simulink model "CAN_TX_RX"  (R2020a)
settings: Solver=FixedStepDiscrete  StartTime=0.0  StopTime=10.0  FixedStep=50e-3  RelTol=1e-3  EnableMultiTasking=on
InitFcn:
  | mbd_s32k_consistency_checks(bdroot(gcs));
undefined symbols (not defined in the file or in its folder): Data, LQFP
libraries: mbd_s32k1xx_ec_toolbox x40, simulink x17, etargetslib x15
(part 1 of 2)
settings Model: Creator=RolandoA  LastModifiedBy=rolan
settings DataIOCC: ExternalInput=off  InitialState=off  SaveOutput=off  SignalLogging=off  SaveTime=off
settings OptimizationCC: DefaultParameterBehavior=Inlined  EnhancedBackFolding=on  PassReuseOutputArgsAs=Individual arguments  ZeroExternalMemoryAtStartup=off  ZeroInternalMemoryAtStartup=off  OptimizeBlockOrder=speed  DifferentSizesBufferReuse=on  OptimizationCustomize=off  EfficientTunableParamExpr=on
settings DebuggingCC: InheritedTsInSrcMsg=none  SingleTaskRateTransMsg=error  ParameterTunabilityLossMsg=error  UnconnectedInputMsg=error  UnconnectedOutputMsg=error  UnconnectedLineMsg=error  UnknownTsInhSupMsg=error
settings HardwareCC: ProdBitPerPointer=32  ProdBitPerSizeT=32  ProdBitPerPtrDiffT=32  ProdLargestAtomicInteger=Long  ProdLargestAtomicFloat=Double  ProdWordSize=32  ProdHWDeviceType=ARM Compatible->ARM Cortex
settings SFSimCC: MATLABDynamicMemAlloc=off
settings RTWCC: Description=Model Based Design Toolbox S32K1xx Code Generation Target  SystemTargetFile=mbd_s32k.tlc  MakeCommand=mbd_s32k_make_rtw COPY_MDLREF_INCLUDES=0  TemplateMakefile=mbd_s32k.tmf  GenerateReport=on  IncludeHyperlinkInReport=on  LaunchReport=on  GenerateTraceInfo=on  GenerateTraceReport=on  GenerateTraceReportSl=on  GenerateTraceReportSf=on  GenerateTraceReportEml=on  GenerateCodeMetricsReport=on  GenerateCodeReplacementReport=on
settings CodeAppCC: ForceParamTrailComments=on  IgnoreCustomStorageClasses=off  OperatorAnnotations=on  SimulinkDataObjDesc=on  SFDataObjDesc=on  InsertBlockDesc=on
settings STFCustomTargetCC: TargetLangStandard=C99 (ISO)  MultiwordLength=256  CombineOutputUpdateFcns=on  ERTCustomFileBanners=on  SupportContinuousTime=off  SupportNonInlinedSFcns=off  RemoveResetFunc=on  MATLABClassNameForMDSCustomization=Simulink.SoftwareTarget.ERTCustomization  SystemTargetFile=mbd_s32k.tlc
settings ERTTargetCC: TargetLangStandard=C99 (ISO)  ParMdlRefBuildCompliant=off  CompOptLevelCompliant=off  ConcurrentExecutionCompliant=off  ModelStepFunctionPrototypeControlCompliant=off  CPPClassGenCompliant=off  UseToolchainInfoCompliant=off  InlinedParameterPlacement=NonHierarchical  ERTSrcFileBannerTemplate=mbd_ert_code_template.cgt  ERTHdrFileBannerTemplate=mbd_ert_code_template.cgt  ERTDataSrcFileTemplate=mbd_ert_code_template.cgt  ERTDataHdrFileTemplate=mbd_ert_code_template.cgt  ERTCustomFileTemplate=example_file_process.tlc

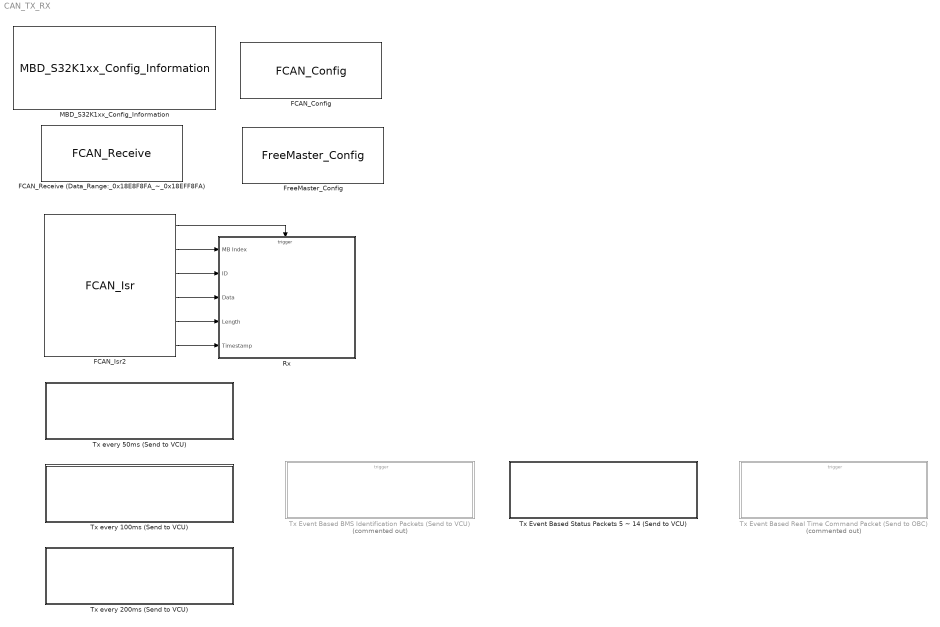
== system CAN_TX_RX ==
  FCAN_Config : mbd_s32k1xx_ec_toolbox/Communication Blocks/CAN Blocks/FCAN_Config  Priority=1  can_instance=0  can_mode=Normal mode  can_max_num_mb=32  can_rx=PTE4: [CAN0_RX | CAN Rx channel]  can_tx=PTE5: [CAN0_TX | CAN Tx Channel]  show_adv_opts=on  can_clk_src=Peripheral clock  bitrate=250  bitrate_adv_opts=off  can_presdiv=15  can_rjw=3  can_pseg1=6  can_pseg2=3  can_propseg=7  can_cbt_presdiv=39  can_cbt_rjw=3  can_cbt_pseg1=5  can_cbt_pseg2=5  can_cbt_propseg=27  can_fd_enable=off  can_payload=8  can_rxfifo_enable=off  can_fifo_id_filter_extended=on  can_fifo_id_filter_remote=off  can_num_id_filters=8  can_fifo_id_format=A  can_fifo_id_filter={'0x0', '0x0', '0x0', '0x0', '0x0', '0x0', '0x0', '0x0'}  can_pn_enable=off  can_wakeup_match=off  can_wakeup_timeout=off  can_timeout_en=off  can_match_timeout=1  can_multiple_matches_en=off  can_num_matches=1  can_idfilter_extendedid=off  can_idfilter_remoteframe=off  can_idfilter_type=Match exact  can_idfilter_id1=0  can_idfilter_id2=0  can_payloadfilter_enable=off  can_payloadfilter_dlclow=0  can_payloadfilter_dlchigh=0  can_payloadfilter_type=Match exact  can_payloadfilter_payload1_b0=0  can_payloadfilter_payload1_b1=0  can_payloadfilter_payload1_b2=0  can_payloadfilter_payload1_b3=0  can_payloadfilter_payload1_b4=0  can_payloadfilter_payload1_b5=0  can_payloadfilter_payload1_b6=0  can_payloadfilter_payload1_b7=0  can_payloadfilter_payload2_b0=0  can_payloadfilter_payload2_b1=0  can_payloadfilter_payload2_b2=0  can_payloadfilter_payload2_b3=0  can_payloadfilter_payload2_b4=0  can_payloadfilter_payload2_b5=0  can_payloadfilter_payload2_b6=0  can_payloadfilter_payload2_b7=0
  FCAN_Isr2 : mbd_s32k1xx_ec_toolbox/Communication Blocks/CAN Blocks/FCAN_Isr  can_instance=0  can_event=Rx Complete
  FCAN_Receive (Data_Range:_0x18E8F8FA_~_0x18EFF8FA) : mbd_s32k1xx_ec_toolbox/Communication Blocks/CAN Blocks/FCAN_Receive  can_instance=0  can_mode=Non-blocking  can_timeout_ms=0  can_mb_idx=0  can_extended_id=on  can_is_remote=off  can_id=18E8F8FA  can_msg_mask=FFF8FFFF  show_adv_opts=on  can_use_rxfifo=off  can_fd_enable=off
  FreeMaster_Config : mbd_s32k1xx_ec_toolbox/Utility Blocks/FreeMaster_Config  interface=LPUART1  baudrate=115200  rxd=PTC6: [LPUART1_RX | Receive]  txd=PTC7: [LPUART1_TX | Transmit]  mode=Poll-driven  isr_prio=15  show_adv_opts=on  use_scope=on  max_scope_vars=8  use_recorder=on  max_rec_vars=8  rec_buff_size=1024  rec_timebase=0 seconds  comm_buffer_size_auto=on  comm_buffer_size=255  comm_rqueue_size_default=on  comm_rqueue_size=32
  MBD_S32K1xx_Config_Information : mbd_s32k1xx_ec_toolbox/MBD_S32K1xx_Config_Information  mbdt_ver=0  disp_str=|  config_params=[]  mcu_target_name=S32K144  mcu_target_package=100-LQFP  mcu_target_sram_size=64KB  mcu_system_clock_freq=80  mcu_xtal_freq=External 8  mcu_steptick_timer=LPIT Channel 0  mcu_steptick_prio=15  ds_import_enable=on  target_compiler=GCC  target_memory=FLASH  gcc_target_compile_opts=-mthumb -mfloat-abi=hard -mfpu=fpv4-sp-d16 -O1 -g -gstrict-dwarf  gcc_target_assemble_opts=-mthumb -mfloat-abi=hard -mfpu=fpv4-sp-d16 -g  gcc_target_link_opts=-mthumb -mfloat-abi=hard -mfpu=fpv4-sp-d16  gcc_target_default_lcf=on  gcc_target_user_lcf=S32K148_192_flash.ld  ghs_target_compile_opts=-cpu=cortexm4f -thumb -fpu=vfpv4_d16 -fsingle -Ogeneral -Wundef -Wimplicit-int -Wshadow -Wtrigraphs --no_commons --gnu_asm -gnu99 -gdwarf-2 -G  ghs_target_assemble_opts=-cpu=cortexm4f -fpu=vfpv4_d16  ghs_target_link_opts=-cpu=cortexm4f -thumb -fpu=vfpv4_d16  ghs_target_default_lcf=on  ghs_target_user_lcf=S32K148_192_flash.ld  iar_target_compile_opts=--cpu=Cortex-M4F --thumb --fpu=VFPv4_sp -Ol -e --debug --dlib_config normal  iar_target_assemble_opts=--cpu Cortex-M4F --thumb --fpu VFPv4_sp  iar_target_link_opts=--no_exceptions --vfe --inline  iar_target_default_lcf=on  iar_target_user_lcf=S32K148_192_flash.icf  pil_download_enable=off  rbl_download_enable=on  rbl_start_delay=5000  rbl_download_interface=OpenSDA  rbl_restart_request=off  rbl_com_port=Custom  rbl_com_port_custom=COM1  pil_download_rate=57600  pil_opensda_drive=Custom  pil_opensda_drive_custom=D  pil_uart_instance=1  pil_uart_rx=PTC6: [LPUART1_RX | Receive]  pil_uart_tx=PTC7: [LPUART1_TX | Transmit]  FTM_PWM_PcrCheckEnDis=on  FTM_Input_Edge_Inputs_PcrCheckEnDis=on  FTM_Dual_Edge_Inputs_PcrCheckEnDis=on  FTM_Quadrature_Inputs_PcrCheckEnDis=on  FTM_Hall_Sensor_Inputs_PcrCheckEnDis=on  LPTMR_PcrCheckEnDis=on  PIT_PcrCheckEnDis=on  RTC_PcrCheckEnDis=on  FlexCAN_PcrCheckEnDis=on  LIN_PcrCheckEnDis=on  FlexIO_PcrCheckEnDis=on  LPI2C_PcrCheckEnDis=on  LPSPI_PcrCheckEnDis=on  LPUART_PcrCheckEnDis=on  CMP_PcrCheckEnDis=on  GPIO_OutputPcrCheckEnDis=on  GPIO_InputPcrCheckEnDis=on  SBC_PcrCheckEnDis=on  BMS_PcrCheckEnDis=on  AMMCLIB_PcrCheckEnDis=on  FM_PcrCheckEnDis=on  Profile_PcrCheckEnDis=on  ConfigParams_PcrCheckEnDis=on  ModelRef_PcrCheckEnDis=on  PDB0_PcrCheckEnDis=on  CSEc_PcrCheckEnDis=on  eDMA_PcrCheckEnDis=on  FLASH_PcrCheckEnDis=on  ADC_PcrCheckEnDis=on  WDOG_PcrCheckEnDis=on
      | Target : S32K144-64KB_SRAM
      | Package : 100-pin
      | System clock : 80 MHz
      | XTAL clock : External 8 MHz
      | Compiler : IAR
      | Target Type : FLASH
      | Download Code after build : off
      | Step Tick Interrupt Priority : 15
  Rx : Subsystem  TreatAsAtomicUnit=on
  "Tx Event Based BMS Identification Packets (Send to VCU)   " : Subsystem  Commented=on  TreatAsAtomicUnit=on
  Tx Event Based Real Time Command Packet (Send to OBC) : Subsystem  Commented=on  TreatAsAtomicUnit=on
  Tx Event Based Status Packets 5 ~ 14 (Send to VCU) : Subsystem  TreatAsAtomicUnit=on
  Tx every 100ms (Send to VCU) : Subsystem  TreatAsAtomicUnit=on  SystemSampleTime=100e-3
  Tx every 200ms (Send to VCU) : Subsystem  TreatAsAtomicUnit=on  SystemSampleTime=200e-3
  Tx every 50ms (Send to VCU) : Subsystem  TreatAsAtomicUnit=on  SystemSampleTime=50e-3
  wires:
  FCAN_Isr2/1 -> Rx/Trigger
  FCAN_Isr2/2 -> Rx/1(MB Index)
  FCAN_Isr2/3 -> Rx/2(ID)
  FCAN_Isr2/4 -> Rx/3(Data)
  FCAN_Isr2/5 -> Rx/4(Length)
  FCAN_Isr2/6 -> Rx/5(Timestamp)

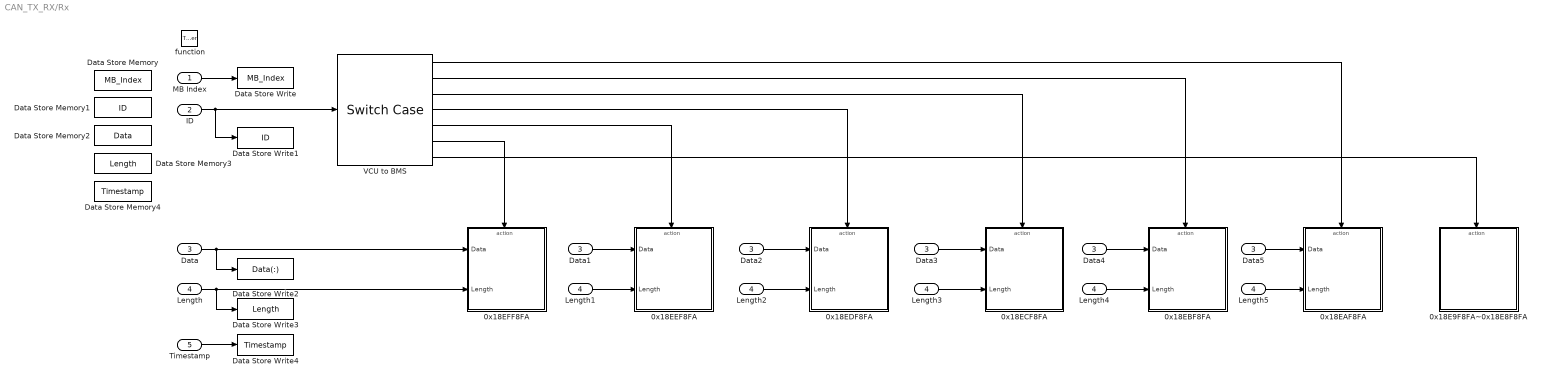
== system CAN_TX_RX/Rx ==
  MB Index : Inport
  ID : Inport  Port=2
  Data : Inport  Port=3
  Length : Inport  Port=4
  Timestamp : Inport  Port=5
  function : TriggerPort  TriggerType=function-call  VariantControl=Variant
  0x18E9F8FA~0x18E8F8FA : Subsystem  TreatAsAtomicUnit=on
  0x18EAF8FA : Subsystem  TreatAsAtomicUnit=on
  0x18EBF8FA : Subsystem  TreatAsAtomicUnit=on
  0x18ECF8FA : Subsystem  TreatAsAtomicUnit=on
  0x18EDF8FA : Subsystem  TreatAsAtomicUnit=on
  0x18EEF8FA : Subsystem  TreatAsAtomicUnit=on
  0x18EFF8FA : Subsystem  TreatAsAtomicUnit=on
  Data Store Memory : DataStoreMemory  DataStoreName=MB_Index  ReadBeforeWriteMsg=warning  WriteAfterWriteMsg=warning  WriteAfterReadMsg=warning  ShowAdditionalParam=off  OutDataTypeStr=uint8
  Data Store Memory1 : DataStoreMemory  DataStoreName=ID  ReadBeforeWriteMsg=warning  WriteAfterWriteMsg=warning  WriteAfterReadMsg=warning  ShowAdditionalParam=off  OutDataTypeStr=uint32
  Data Store Memory2 : DataStoreMemory  DataStoreName=Data  ReadBeforeWriteMsg=warning  WriteAfterWriteMsg=warning  WriteAfterReadMsg=warning  InitialValue=[0 0 0 0 0 0 0 0]  ShowAdditionalParam=off  OutDataTypeStr=uint8
  Data Store Memory3 : DataStoreMemory  DataStoreName=Length  ReadBeforeWriteMsg=warning  WriteAfterWriteMsg=warning  WriteAfterReadMsg=warning  ShowAdditionalParam=off  OutDataTypeStr=uint8
  Data Store Memory4 : DataStoreMemory  DataStoreName=Timestamp  ReadBeforeWriteMsg=warning  WriteAfterWriteMsg=warning  WriteAfterReadMsg=warning  ShowAdditionalParam=off  OutDataTypeStr=uint16
  Data Store Write : DataStoreWrite  DataStoreName=MB_Index
  Data Store Write1 : DataStoreWrite  DataStoreName=ID
  Data Store Write2 : DataStoreWrite  DataStoreName=Data  DataStoreElements=Data(:)
  Data Store Write3 : DataStoreWrite  DataStoreName=Length
  Data Store Write4 : DataStoreWrite  DataStoreName=Timestamp
  Data{1..5} (5 alike) : InportShadow  Port=3
  Length{1..5} (5 alike) : InportShadow  Port=4
  VCU to BMS : SwitchCase  CaseConditions={418052346, 418117882, 418183418, 418248954, 418314490, 418380026}
  wires:
  MB Index/1 -> Data Store Write/1
  ID/1 -> VCU to BMS/1, Data Store Write1/1
  Data/1 -> Data Store Write2/1, 0x18EFF8FA/1(Data)
  Length/1 -> Data Store Write3/1, 0x18EFF8FA/2(Length)
  Timestamp/1 -> Data Store Write4/1
  VCU to BMS/7 -> 0x18E9F8FA~0x18E8F8FA/Action
  VCU to BMS/6 -> 0x18EFF8FA/Action
  VCU to BMS/2 -> 0x18EBF8FA/Action
  VCU to BMS/3 -> 0x18ECF8FA/Action
  VCU to BMS/4 -> 0x18EDF8FA/Action
  VCU to BMS/5 -> 0x18EEF8FA/Action
  Data1/1 -> 0x18EEF8FA/1(Data)
  Length1/1 -> 0x18EEF8FA/2(Length)
  Data2/1 -> 0x18EDF8FA/1(Data)
  Length2/1 -> 0x18EDF8FA/2(Length)
  Length3/1 -> 0x18ECF8FA/2(Length)
  Data3/1 -> 0x18ECF8FA/1(Data)
  Data4/1 -> 0x18EBF8FA/1(Data)
  Length4/1 -> 0x18EBF8FA/2(Length)
  VCU to BMS/1 -> 0x18EAF8FA/Action
  Data5/1 -> 0x18EAF8FA/1(Data)
  Length5/1 -> 0x18EAF8FA/2(Length)

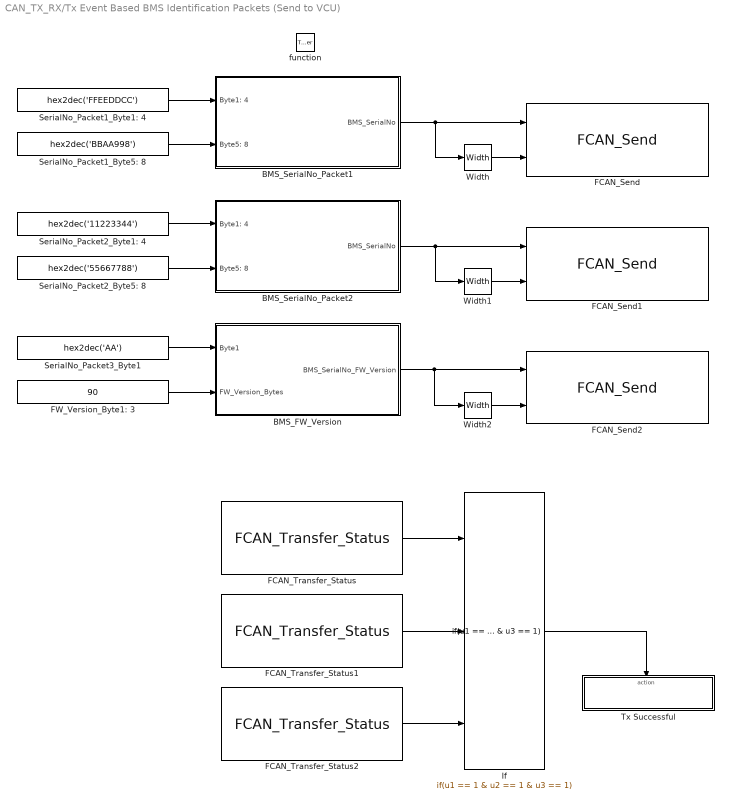
== system CAN_TX_RX/Tx Event Based BMS Identification Packets (Send to VCU)    ==
  function : TriggerPort  TriggerType=function-call  VariantControl=Variant
  BMS_FW_Version : Subsystem
  BMS_SerialNo_Packet1 : Subsystem
  BMS_SerialNo_Packet2 : Subsystem
  FCAN_Send : mbd_s32k1xx_ec_toolbox/Communication Blocks/CAN Blocks/FCAN_Send  can_instance=0  can_mode=Non-blocking  can_timeout_ms=0  can_mb_idx=5  can_extended_id=on  can_is_remote=off  can_id=18EBFAF8  show_adv_opts=on  can_fd_enable=off  can_enable_brs=off  can_fd_padding=0
  FCAN_Send1 : mbd_s32k1xx_ec_toolbox/Communication Blocks/CAN Blocks/FCAN_Send  can_instance=0  can_mode=Non-blocking  can_timeout_ms=0  can_mb_idx=6  can_extended_id=on  can_is_remote=off  can_id=18EAFAF8  show_adv_opts=on  can_fd_enable=off  can_enable_brs=off  can_fd_padding=0
  FCAN_Send2 : mbd_s32k1xx_ec_toolbox/Communication Blocks/CAN Blocks/FCAN_Send  can_instance=0  can_mode=Non-blocking  can_timeout_ms=0  can_mb_idx=7  can_extended_id=on  can_is_remote=off  can_id=18E9FAF8  show_adv_opts=on  can_fd_enable=off  can_enable_brs=off  can_fd_padding=0
  FCAN_Transfer_Status : mbd_s32k1xx_ec_toolbox/Communication Blocks/CAN Blocks/FCAN_Transfer_Status  can_instance=0  can_mb_idx=5
  FCAN_Transfer_Status1 : mbd_s32k1xx_ec_toolbox/Communication Blocks/CAN Blocks/FCAN_Transfer_Status  can_instance=0  can_mb_idx=6
  FCAN_Transfer_Status2 : mbd_s32k1xx_ec_toolbox/Communication Blocks/CAN Blocks/FCAN_Transfer_Status  can_instance=0  can_mb_idx=7
  FW_Version_Byte1: 3 : Constant  Value=90  OutDataTypeStr=uint32
  If : If  NumInputs=3  IfExpression=u1 == 1 & u2 == 1 & u3 == 1  ShowElse=off
  SerialNo_Packet1_Byte1: 4 : Constant  Value=hex2dec('FFEEDDCC')  OutDataTypeStr=uint32
  SerialNo_Packet1_Byte5: 8 : Constant  Value=hex2dec('BBAA998')  OutDataTypeStr=uint32
  SerialNo_Packet2_Byte1: 4 : Constant  Value=hex2dec('11223344')  OutDataTypeStr=uint32
  SerialNo_Packet2_Byte5: 8 : Constant  Value=hex2dec('55667788')  OutDataTypeStr=uint32
  SerialNo_Packet3_Byte1 : Constant  Value=hex2dec('AA')  OutDataTypeStr=uint8
  Tx Successful : Subsystem  TreatAsAtomicUnit=on
  Width : Width  DataType=uint8
  Width1 : Width  DataType=uint8
  Width2 : Width  DataType=uint8
  wires:
  BMS_SerialNo_Packet1/1(BMS_SerialNo) -> Width/1, FCAN_Send/1
  Width/1 -> FCAN_Send/2
  FCAN_Transfer_Status/1 -> If/1
  FCAN_Transfer_Status1/1 -> If/2
  FCAN_Transfer_Status2/1 -> If/3
  If/1 -> Tx Successful/Action
  Width1/1 -> FCAN_Send1/2
  Width2/1 -> FCAN_Send2/2
  SerialNo_Packet1_Byte1: 4/1 -> BMS_SerialNo_Packet1/1(Byte1: 4)
  SerialNo_Packet1_Byte5: 8/1 -> BMS_SerialNo_Packet1/2(Byte5: 8)
  SerialNo_Packet2_Byte1: 4/1 -> BMS_SerialNo_Packet2/1(Byte1: 4)
  SerialNo_Packet2_Byte5: 8/1 -> BMS_SerialNo_Packet2/2(Byte5: 8)
  BMS_SerialNo_Packet2/1(BMS_SerialNo) -> Width1/1, FCAN_Send1/1
  SerialNo_Packet3_Byte1/1 -> BMS_FW_Version/1(Byte1)
  FW_Version_Byte1: 3/1 -> BMS_FW_Version/2(FW_Version_Bytes)
  BMS_FW_Version/1(BMS_SerialNo_FW_Version) -> Width2/1, FCAN_Send2/1

== system CAN_TX_RX/Tx Event Based Real Time Command Packet (Send to OBC) ==
  function : TriggerPort  TriggerType=function-call  VariantControl=Variant
  FCAN_Send : mbd_s32k1xx_ec_toolbox/Communication Blocks/CAN Blocks/FCAN_Send  Commented=on  can_instance=0  can_mode=Non-blocking  can_timeout_ms=0  can_mb_idx=18  can_extended_id=on  can_is_remote=off  can_id=18EFF2F8  show_adv_opts=on  can_fd_enable=off  can_enable_brs=off  can_fd_padding=0
  FCAN_Transfer_Status : mbd_s32k1xx_ec_toolbox/Communication Blocks/CAN Blocks/FCAN_Transfer_Status  Commented=on  can_instance=0  can_mb_idx=18
  If : If  Commented=on  IfExpression=u1 == 1  ShowElse=off
  Tx Successful : Subsystem  Commented=on  TreatAsAtomicUnit=on
  wires:
  FCAN_Transfer_Status/1 -> If/1
  If/1 -> Tx Successful/Action

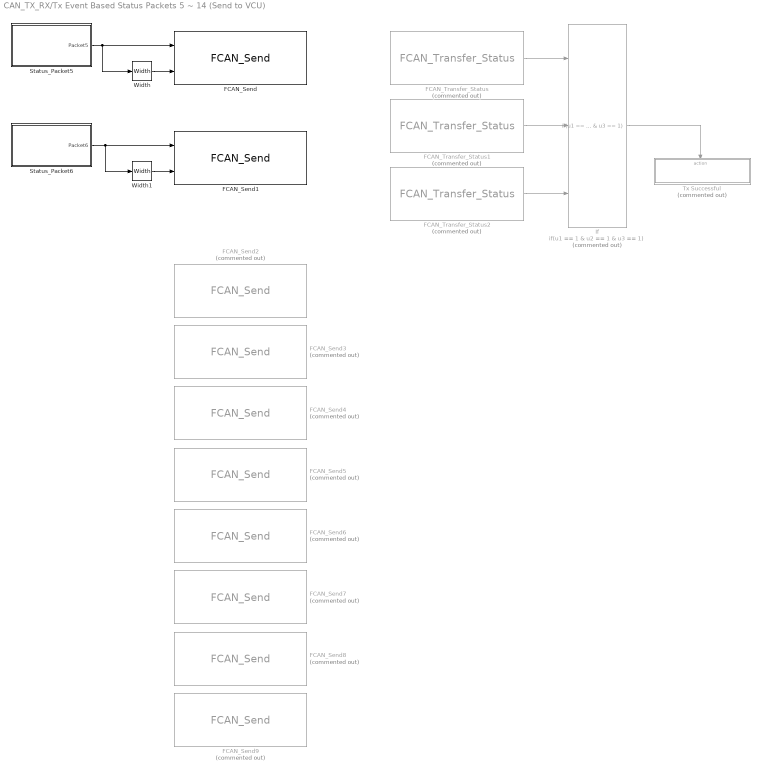
== system CAN_TX_RX/Tx Event Based Status Packets 5 ~ 14 (Send to VCU) ==
  FCAN_Send : mbd_s32k1xx_ec_toolbox/Communication Blocks/CAN Blocks/FCAN_Send  can_instance=0  can_mode=Non-blocking  can_timeout_ms=0  can_mb_idx=8  can_extended_id=on  can_is_remote=off  can_id=18E8FAF8  show_adv_opts=on  can_fd_enable=off  can_enable_brs=off  can_fd_padding=0
  FCAN_Send1 : mbd_s32k1xx_ec_toolbox/Communication Blocks/CAN Blocks/FCAN_Send  can_instance=0  can_mode=Non-blocking  can_timeout_ms=0  can_mb_idx=9  can_extended_id=on  can_is_remote=off  can_id=18E7FAF8  show_adv_opts=on  can_fd_enable=off  can_enable_brs=off  can_fd_padding=0
  FCAN_Send2 : mbd_s32k1xx_ec_toolbox/Communication Blocks/CAN Blocks/FCAN_Send  Commented=on  can_instance=0  can_mode=Non-blocking  can_timeout_ms=0  can_mb_idx=10  can_extended_id=on  can_is_remote=off  can_id=18E6FAF8  show_adv_opts=on  can_fd_enable=off  can_enable_brs=off  can_fd_padding=0
  FCAN_Send3 : mbd_s32k1xx_ec_toolbox/Communication Blocks/CAN Blocks/FCAN_Send  Commented=on  can_instance=0  can_mode=Non-blocking  can_timeout_ms=0  can_mb_idx=11  can_extended_id=on  can_is_remote=off  can_id=18E5FAF8  show_adv_opts=on  can_fd_enable=off  can_enable_brs=off  can_fd_padding=0
  FCAN_Send4 : mbd_s32k1xx_ec_toolbox/Communication Blocks/CAN Blocks/FCAN_Send  Commented=on  can_instance=0  can_mode=Non-blocking  can_timeout_ms=0  can_mb_idx=12  can_extended_id=on  can_is_remote=off  can_id=18E4FAF8  show_adv_opts=on  can_fd_enable=off  can_enable_brs=off  can_fd_padding=0
  FCAN_Send5 : mbd_s32k1xx_ec_toolbox/Communication Blocks/CAN Blocks/FCAN_Send  Commented=on  can_instance=0  can_mode=Non-blocking  can_timeout_ms=0  can_mb_idx=13  can_extended_id=on  can_is_remote=off  can_id=18E3FAF8  show_adv_opts=on  can_fd_enable=off  can_enable_brs=off  can_fd_padding=0
  FCAN_Send6 : mbd_s32k1xx_ec_toolbox/Communication Blocks/CAN Blocks/FCAN_Send  Commented=on  can_instance=0  can_mode=Non-blocking  can_timeout_ms=0  can_mb_idx=14  can_extended_id=on  can_is_remote=off  can_id=18E2FAF8  show_adv_opts=on  can_fd_enable=off  can_enable_brs=off  can_fd_padding=0
  FCAN_Send7 : mbd_s32k1xx_ec_toolbox/Communication Blocks/CAN Blocks/FCAN_Send  Commented=on  can_instance=0  can_mode=Non-blocking  can_timeout_ms=0  can_mb_idx=15  can_extended_id=on  can_is_remote=off  can_id=18E1FAF8  show_adv_opts=on  can_fd_enable=off  can_enable_brs=off  can_fd_padding=0
  FCAN_Send8 : mbd_s32k1xx_ec_toolbox/Communication Blocks/CAN Blocks/FCAN_Send  Commented=on  can_instance=0  can_mode=Non-blocking  can_timeout_ms=0  can_mb_idx=16  can_extended_id=on  can_is_remote=off  can_id=18E0FAF8  show_adv_opts=on  can_fd_enable=off  can_enable_brs=off  can_fd_padding=0
  FCAN_Send9 : mbd_s32k1xx_ec_toolbox/Communication Blocks/CAN Blocks/FCAN_Send  Commented=on  can_instance=0  can_mode=Non-blocking  can_timeout_ms=0  can_mb_idx=17  can_extended_id=on  can_is_remote=off  can_id=18DFFAF8  show_adv_opts=on  can_fd_enable=off  can_enable_brs=off  can_fd_padding=0
  FCAN_Transfer_Status : mbd_s32k1xx_ec_toolbox/Communication Blocks/CAN Blocks/FCAN_Transfer_Status  Commented=on  can_instance=0  can_mb_idx=5
  FCAN_Transfer_Status1 : mbd_s32k1xx_ec_toolbox/Communication Blocks/CAN Blocks/FCAN_Transfer_Status  Commented=on  can_instance=0  can_mb_idx=6
  FCAN_Transfer_Status2 : mbd_s32k1xx_ec_toolbox/Communication Blocks/CAN Blocks/FCAN_Transfer_Status  Commented=on  can_instance=0  can_mb_idx=7
  If : If  Commented=on  NumInputs=3  IfExpression=u1 == 1 & u2 == 1 & u3 == 1  ShowElse=off
  Status_Packet5 : Subsystem
  Status_Packet6 : Subsystem
  Tx Successful : Subsystem  Commented=on  TreatAsAtomicUnit=on
  Width : Width  DataType=uint8
  Width1 : Width  DataType=uint8
  wires:
  If/1 -> Tx Successful/Action
  FCAN_Transfer_Status2/1 -> If/3
  FCAN_Transfer_Status1/1 -> If/2
  FCAN_Transfer_Status/1 -> If/1
  Status_Packet5/1(Packet5) -> FCAN_Send/1, Width/1
  Width/1 -> FCAN_Send/2
  Width1/1 -> FCAN_Send1/2
  Status_Packet6/1(Packet6) -> Width1/1, FCAN_Send1/1

== system CAN_TX_RX/Tx every 100ms (Send to VCU) ==
  FCAN_Send : mbd_s32k1xx_ec_toolbox/Communication Blocks/CAN Blocks/FCAN_Send  can_instance=0  can_mode=Non-blocking  can_timeout_ms=0  can_mb_idx=4  can_extended_id=on  can_is_remote=off  can_id=18ECFAF8  show_adv_opts=on  can_fd_enable=off  can_enable_brs=off  can_fd_padding=0
  FCAN_Transfer_Status : mbd_s32k1xx_ec_toolbox/Communication Blocks/CAN Blocks/FCAN_Transfer_Status  can_instance=0  can_mb_idx=4
  If : If  IfExpression=u1 == 1  ShowElse=off
  Status_Packet4 : Subsystem
  Tx Succesful : Subsystem  TreatAsAtomicUnit=on
  Width : Width  DataType=uint8
  wires:
  Width/1 -> FCAN_Send/2
  Status_Packet4/1(Packet4) -> FCAN_Send/1, Width/1
  If/1 -> Tx Succesful/Action
  FCAN_Transfer_Status/1 -> If/1

== system CAN_TX_RX/Tx every 200ms (Send to VCU) ==
  FCAN_Send : mbd_s32k1xx_ec_toolbox/Communication Blocks/CAN Blocks/FCAN_Send  can_instance=0  can_mode=Non-blocking  can_timeout_ms=0  can_mb_idx=2  can_extended_id=on  can_is_remote=off  can_id=18EEFAF8  show_adv_opts=on  can_fd_enable=off  can_enable_brs=off  can_fd_padding=0
  FCAN_Send1 : mbd_s32k1xx_ec_toolbox/Communication Blocks/CAN Blocks/FCAN_Send  can_instance=0  can_mode=Non-blocking  can_timeout_ms=0  can_mb_idx=3  can_extended_id=on  can_is_remote=off  can_id=18EDFAF8  show_adv_opts=on  can_fd_enable=off  can_enable_brs=off  can_fd_padding=0
  FCAN_Transfer_Status : mbd_s32k1xx_ec_toolbox/Communication Blocks/CAN Blocks/FCAN_Transfer_Status  can_instance=0  can_mb_idx=2
  FCAN_Transfer_Status1 : mbd_s32k1xx_ec_toolbox/Communication Blocks/CAN Blocks/FCAN_Transfer_Status  can_instance=0  can_mb_idx=3
  If : If  NumInputs=2  IfExpression=u1 == 1 & u2 == 1  ShowElse=off
  Status_Packet2 : Subsystem
  Status_Packet3 : Subsystem
  Tx Successful : Subsystem  TreatAsAtomicUnit=on
  Width : Width  DataType=uint8
  Width1 : Width  DataType=uint8
  wires:
  Width/1 -> FCAN_Send/2
  Status_Packet2/1(Packet2) -> FCAN_Send/1, Width/1
  If/1 -> Tx Successful/Action
  FCAN_Transfer_Status/1 -> If/1
  Width1/1 -> FCAN_Send1/2
  Status_Packet3/1(Packet3) -> Width1/1, FCAN_Send1/1
  FCAN_Transfer_Status1/1 -> If/2

== system CAN_TX_RX/Tx every 50ms (Send to VCU) ==
  FCAN_Send : mbd_s32k1xx_ec_toolbox/Communication Blocks/CAN Blocks/FCAN_Send  can_instance=0  can_mode=Non-blocking  can_timeout_ms=0  can_mb_idx=1  can_extended_id=on  can_is_remote=off  can_id=18EFFAF8  show_adv_opts=on  can_fd_enable=off  can_enable_brs=off  can_fd_padding=0
  FCAN_Transfer_Status : mbd_s32k1xx_ec_toolbox/Communication Blocks/CAN Blocks/FCAN_Transfer_Status  can_instance=0  can_mb_idx=1
  If : If  IfExpression=u1 == 1  ShowElse=off
  Status_Packet1 : Subsystem
  Tx Succesful : Subsystem  TreatAsAtomicUnit=on
  Width : Width  DataType=uint8
  wires:
  FCAN_Transfer_Status/1 -> If/1
  If/1 -> Tx Succesful/Action
  Status_Packet1/1(Packet1) -> Width/1, FCAN_Send/1
  Width/1 -> FCAN_Send/2

== system CAN_TX_RX/Rx/0x18E9F8FA~0x18E8F8FA ==
  Action Port : ActionPort  ActionPortLabel=default:

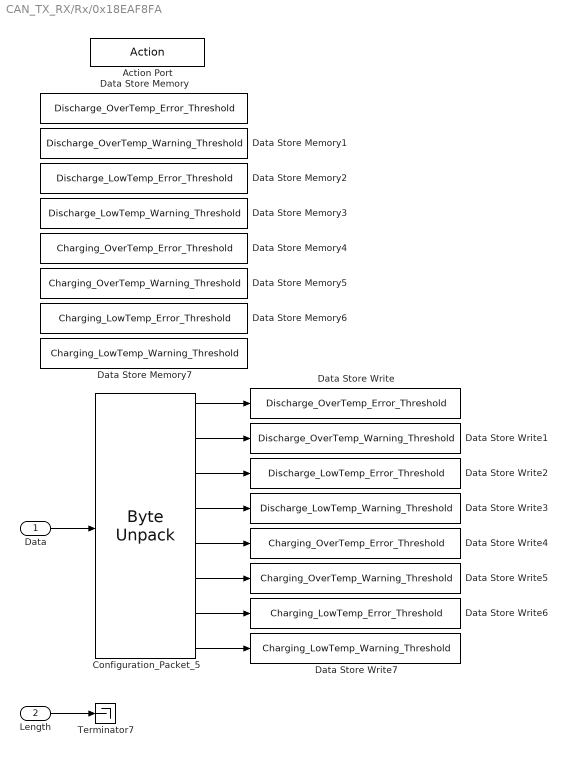
== system CAN_TX_RX/Rx/0x18EAF8FA ==
  Data : Inport
  Length : Inport  Port=2
  Action Port : ActionPort  ActionPortLabel=case [ 418052346 ]:
  Configuration_Packet_5 : etargetslib/Byte Unpack  dimensions={1, 1, 1, 1, 1, 1, 1, 1}  datatypes={'uint8', 'uint8', 'uint8', 'uint8', 'uint8', 'uint8', 'uint8', 'uint8'}  byteAlign=1
  Data Store Memory : DataStoreMemory  DataStoreName=Discharge_OverTemp_Error_Threshold  ReadBeforeWriteMsg=warning  WriteAfterWriteMsg=warning  WriteAfterReadMsg=warning  ShowAdditionalParam=off
  Data Store Memory1 : DataStoreMemory  DataStoreName=Discharge_OverTemp_Warning_Threshold  ReadBeforeWriteMsg=warning  WriteAfterWriteMsg=warning  WriteAfterReadMsg=warning  ShowAdditionalParam=off
  Data Store Memory2 : DataStoreMemory  DataStoreName=Discharge_LowTemp_Error_Threshold  ReadBeforeWriteMsg=warning  WriteAfterWriteMsg=warning  WriteAfterReadMsg=warning  ShowAdditionalParam=off
  Data Store Memory3 : DataStoreMemory  DataStoreName=Discharge_LowTemp_Warning_Threshold  ReadBeforeWriteMsg=warning  WriteAfterWriteMsg=warning  WriteAfterReadMsg=warning  ShowAdditionalParam=off
  Data Store Memory4 : DataStoreMemory  DataStoreName=Charging_OverTemp_Error_Threshold  ReadBeforeWriteMsg=warning  WriteAfterWriteMsg=warning  WriteAfterReadMsg=warning  ShowAdditionalParam=off
  Data Store Memory5 : DataStoreMemory  DataStoreName=Charging_OverTemp_Warning_Threshold  ReadBeforeWriteMsg=warning  WriteAfterWriteMsg=warning  WriteAfterReadMsg=warning  ShowAdditionalParam=off
  Data Store Memory6 : DataStoreMemory  DataStoreName=Charging_LowTemp_Error_Threshold  ReadBeforeWriteMsg=warning  WriteAfterWriteMsg=warning  WriteAfterReadMsg=warning  ShowAdditionalParam=off
  Data Store Memory7 : DataStoreMemory  DataStoreName=Charging_LowTemp_Warning_Threshold  ReadBeforeWriteMsg=warning  WriteAfterWriteMsg=warning  WriteAfterReadMsg=warning  ShowAdditionalParam=off
  Data Store Write : DataStoreWrite  DataStoreName=Discharge_OverTemp_Error_Threshold
  Data Store Write1 : DataStoreWrite  DataStoreName=Discharge_OverTemp_Warning_Threshold
  Data Store Write2 : DataStoreWrite  DataStoreName=Discharge_LowTemp_Error_Threshold
  Data Store Write3 : DataStoreWrite  DataStoreName=Discharge_LowTemp_Warning_Threshold
  Data Store Write4 : DataStoreWrite  DataStoreName=Charging_OverTemp_Error_Threshold
  Data Store Write5 : DataStoreWrite  DataStoreName=Charging_OverTemp_Warning_Threshold
  Data Store Write6 : DataStoreWrite  DataStoreName=Charging_LowTemp_Error_Threshold
  Data Store Write7 : DataStoreWrite  DataStoreName=Charging_LowTemp_Warning_Threshold
  Terminator7 : Terminator
  wires:
  Data/1 -> Configuration_Packet_5/1
  Length/1 -> Terminator7/1
  Configuration_Packet_5/1 -> Data Store Write/1
  Configuration_Packet_5/2 -> Data Store Write1/1
  Configuration_Packet_5/3 -> Data Store Write2/1
  Configuration_Packet_5/4 -> Data Store Write3/1
  Configuration_Packet_5/5 -> Data Store Write4/1
  Configuration_Packet_5/6 -> Data Store Write5/1
  Configuration_Packet_5/7 -> Data Store Write6/1
  Configuration_Packet_5/8 -> Data Store Write7/1

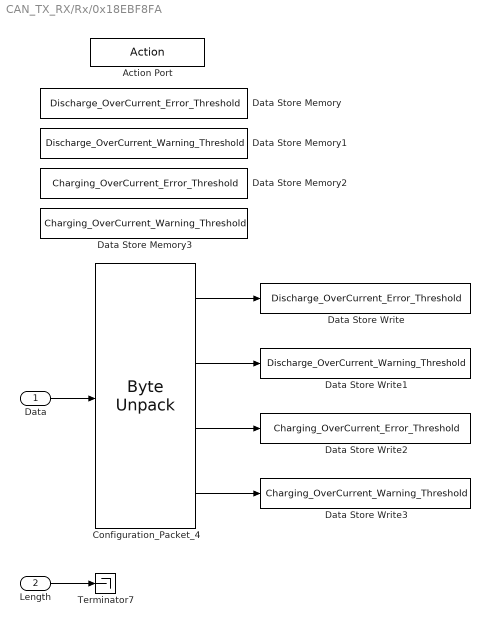
== system CAN_TX_RX/Rx/0x18EBF8FA ==
  Data : Inport
  Length : Inport  Port=2
  Action Port : ActionPort  ActionPortLabel=case [ 418117882 ]:
  Configuration_Packet_4 : etargetslib/Byte Unpack  dimensions={1, 1, 1, 1}  datatypes={'uint16', 'uint16', 'uint16', 'uint16'}  byteAlign=1
  Data Store Memory : DataStoreMemory  DataStoreName=Discharge_OverCurrent_Error_Threshold  ReadBeforeWriteMsg=warning  WriteAfterWriteMsg=warning  WriteAfterReadMsg=warning  ShowAdditionalParam=off
  Data Store Memory1 : DataStoreMemory  DataStoreName=Discharge_OverCurrent_Warning_Threshold  ReadBeforeWriteMsg=warning  WriteAfterWriteMsg=warning  WriteAfterReadMsg=warning  ShowAdditionalParam=off
  Data Store Memory2 : DataStoreMemory  DataStoreName=Charging_OverCurrent_Error_Threshold  ReadBeforeWriteMsg=warning  WriteAfterWriteMsg=warning  WriteAfterReadMsg=warning  ShowAdditionalParam=off
  Data Store Memory3 : DataStoreMemory  DataStoreName=Charging_OverCurrent_Warning_Threshold  ReadBeforeWriteMsg=warning  WriteAfterWriteMsg=warning  WriteAfterReadMsg=warning  ShowAdditionalParam=off
  Data Store Write : DataStoreWrite  DataStoreName=Discharge_OverCurrent_Error_Threshold
  Data Store Write1 : DataStoreWrite  DataStoreName=Discharge_OverCurrent_Warning_Threshold
  Data Store Write2 : DataStoreWrite  DataStoreName=Charging_OverCurrent_Error_Threshold
  Data Store Write3 : DataStoreWrite  DataStoreName=Charging_OverCurrent_Warning_Threshold
  Terminator7 : Terminator
  wires:
  Length/1 -> Terminator7/1
  Data/1 -> Configuration_Packet_4/1
  Configuration_Packet_4/1 -> Data Store Write/1
  Configuration_Packet_4/2 -> Data Store Write1/1
  Configuration_Packet_4/3 -> Data Store Write2/1
  Configuration_Packet_4/4 -> Data Store Write3/1

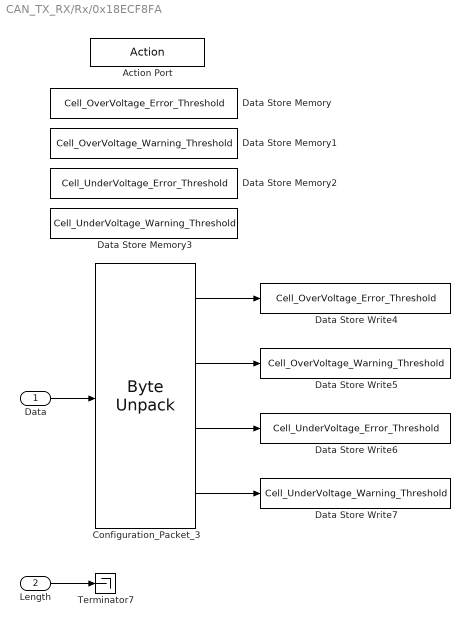
== system CAN_TX_RX/Rx/0x18ECF8FA ==
  Data : Inport
  Length : Inport  Port=2
  Action Port : ActionPort  ActionPortLabel=case [ 418183418 ]:
  Configuration_Packet_3 : etargetslib/Byte Unpack  dimensions={1, 1, 1, 1}  datatypes={'uint16', 'uint16', 'uint16', 'uint16'}  byteAlign=1
  Data Store Memory : DataStoreMemory  DataStoreName=Cell_OverVoltage_Error_Threshold  ReadBeforeWriteMsg=warning  WriteAfterWriteMsg=warning  WriteAfterReadMsg=warning  ShowAdditionalParam=off
  Data Store Memory1 : DataStoreMemory  DataStoreName=Cell_OverVoltage_Warning_Threshold  ReadBeforeWriteMsg=warning  WriteAfterWriteMsg=warning  WriteAfterReadMsg=warning  ShowAdditionalParam=off
  Data Store Memory2 : DataStoreMemory  DataStoreName=Cell_UnderVoltage_Error_Threshold  ReadBeforeWriteMsg=warning  WriteAfterWriteMsg=warning  WriteAfterReadMsg=warning  ShowAdditionalParam=off
  Data Store Memory3 : DataStoreMemory  DataStoreName=Cell_UnderVoltage_Warning_Threshold  ReadBeforeWriteMsg=warning  WriteAfterWriteMsg=warning  WriteAfterReadMsg=warning  ShowAdditionalParam=off
  Data Store Write4 : DataStoreWrite  DataStoreName=Cell_OverVoltage_Error_Threshold
  Data Store Write5 : DataStoreWrite  DataStoreName=Cell_OverVoltage_Warning_Threshold
  Data Store Write6 : DataStoreWrite  DataStoreName=Cell_UnderVoltage_Error_Threshold
  Data Store Write7 : DataStoreWrite  DataStoreName=Cell_UnderVoltage_Warning_Threshold
  Terminator7 : Terminator
  wires:
  Configuration_Packet_3/4 -> Data Store Write7/1
  Configuration_Packet_3/3 -> Data Store Write6/1
  Configuration_Packet_3/2 -> Data Store Write5/1
  Configuration_Packet_3/1 -> Data Store Write4/1
  Data/1 -> Configuration_Packet_3/1
  Length/1 -> Terminator7/1

== system CAN_TX_RX/Rx/0x18EDF8FA ==
  Data : Inport
  Length : Inport  Port=2
  Action Port : ActionPort  ActionPortLabel=case [ 418248954 ]:
  Configuration_Packet_2 : etargetslib/Byte Unpack  dimensions={1, 1, 1, 1}  datatypes={'uint16', 'uint16', 'uint16', 'uint16'}  byteAlign=1
  Data Store Memory : DataStoreMemory  DataStoreName=OverVoltage_Error_Threshold  ReadBeforeWriteMsg=warning  WriteAfterWriteMsg=warning  WriteAfterReadMsg=warning  ShowAdditionalParam=off
  Data Store Memory1 : DataStoreMemory  DataStoreName=OverVoltage_Warning_Threshold  ReadBeforeWriteMsg=warning  WriteAfterWriteMsg=warning  WriteAfterReadMsg=warning  ShowAdditionalParam=off
  Data Store Memory2 : DataStoreMemory  DataStoreName=UnderVoltage_Error_Threshold  ReadBeforeWriteMsg=warning  WriteAfterWriteMsg=warning  WriteAfterReadMsg=warning  ShowAdditionalParam=off
  Data Store Memory3 : DataStoreMemory  DataStoreName=UnderVoltage_Warning_Threshold  ReadBeforeWriteMsg=warning  WriteAfterWriteMsg=warning  WriteAfterReadMsg=warning  ShowAdditionalParam=off
  Data Store Write : DataStoreWrite  DataStoreName=OverVoltage_Error_Threshold
  Data Store Write1 : DataStoreWrite  DataStoreName=OverVoltage_Warning_Threshold
  Data Store Write2 : DataStoreWrite  DataStoreName=UnderVoltage_Error_Threshold
  Data Store Write3 : DataStoreWrite  DataStoreName=UnderVoltage_Warning_Threshold
  Terminator7 : Terminator
  wires:
  Length/1 -> Terminator7/1
  Data/1 -> Configuration_Packet_2/1
  Configuration_Packet_2/1 -> Data Store Write/1
  Configuration_Packet_2/2 -> Data Store Write1/1
  Configuration_Packet_2/3 -> Data Store Write2/1
  Configuration_Packet_2/4 -> Data Store Write3/1

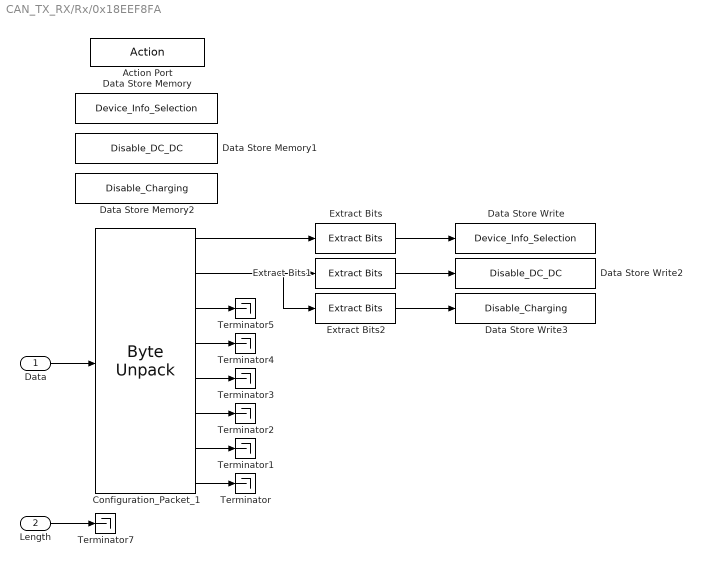
== system CAN_TX_RX/Rx/0x18EEF8FA ==
  Data : Inport
  Length : Inport  Port=2
  Action Port : ActionPort  ActionPortLabel=case [ 418314490 ]:
  Configuration_Packet_1 : etargetslib/Byte Unpack  dimensions={1, 1, 1, 1, 1, 1, 1, 1}  datatypes={'uint8', 'uint8', 'uint8', 'uint8', 'uint8', 'uint8', 'uint8', 'uint8'}  byteAlign=1
  Data Store Memory : DataStoreMemory  DataStoreName=Device_Info_Selection  ReadBeforeWriteMsg=warning  WriteAfterWriteMsg=warning  WriteAfterReadMsg=warning  ShowAdditionalParam=off
  Data Store Memory1 : DataStoreMemory  DataStoreName=Disable_DC_DC  ReadBeforeWriteMsg=warning  WriteAfterWriteMsg=warning  WriteAfterReadMsg=warning  ShowAdditionalParam=off
  Data Store Memory2 : DataStoreMemory  DataStoreName=Disable_Charging  ReadBeforeWriteMsg=warning  WriteAfterWriteMsg=warning  WriteAfterReadMsg=warning  ShowAdditionalParam=off
  Data Store Write : DataStoreWrite  DataStoreName=Device_Info_Selection
  Data Store Write2 : DataStoreWrite  DataStoreName=Disable_DC_DC
  Data Store Write3 : DataStoreWrite  DataStoreName=Disable_Charging
  Extract Bits : simulink/Logic and Bit Operations/Extract Bits  bitsToExtract=Range of bits  numBits=8  bitIdxRange=[0 1]  outScalingMode=Treat bit field as an integer
  Extract Bits1 : simulink/Logic and Bit Operations/Extract Bits  bitsToExtract=Range of bits  numBits=8  bitIdxRange=0  outScalingMode=Treat bit field as an integer
  Extract Bits2 : simulink/Logic and Bit Operations/Extract Bits  bitsToExtract=Range of bits  numBits=8  bitIdxRange=1  outScalingMode=Treat bit field as an integer
  Terminator{,1..5,7} (7 alike) : Terminator
  wires:
  Extract Bits/1 -> Data Store Write/1
  Configuration_Packet_1/1 -> Extract Bits/1
  Data/1 -> Configuration_Packet_1/1
  Length/1 -> Terminator7/1
  Configuration_Packet_1/3 -> Terminator5/1
  Configuration_Packet_1/4 -> Terminator4/1
  Configuration_Packet_1/5 -> Terminator3/1
  Configuration_Packet_1/6 -> Terminator2/1
  Configuration_Packet_1/7 -> Terminator1/1
  Configuration_Packet_1/8 -> Terminator/1
  Extract Bits1/1 -> Data Store Write2/1
  Extract Bits2/1 -> Data Store Write3/1
  Configuration_Packet_1/2 -> Extract Bits2/1, Extract Bits1/1

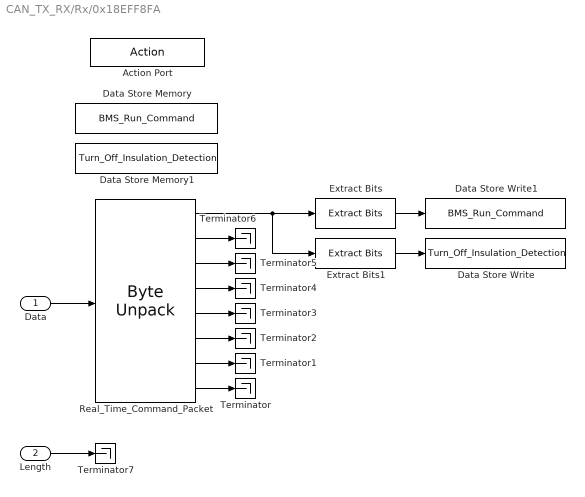
== system CAN_TX_RX/Rx/0x18EFF8FA ==
  Data : Inport
  Length : Inport  Port=2
  Action Port : ActionPort  ActionPortLabel=case [ 418380026 ]:
  Data Store Memory : DataStoreMemory  DataStoreName=BMS_Run_Command  ReadBeforeWriteMsg=warning  WriteAfterWriteMsg=warning  WriteAfterReadMsg=warning  ShowAdditionalParam=off
  Data Store Memory1 : DataStoreMemory  DataStoreName=Turn_Off_Insulation_Detection  ReadBeforeWriteMsg=warning  WriteAfterWriteMsg=warning  WriteAfterReadMsg=warning  ShowAdditionalParam=off
  Data Store Write : DataStoreWrite  DataStoreName=Turn_Off_Insulation_Detection
  Data Store Write1 : DataStoreWrite  DataStoreName=BMS_Run_Command
  Extract Bits : simulink/Logic and Bit Operations/Extract Bits  bitsToExtract=Range of bits  numBits=8  bitIdxRange=[0]  outScalingMode=Treat bit field as an integer
  Extract Bits1 : simulink/Logic and Bit Operations/Extract Bits  bitsToExtract=Range of bits  numBits=8  bitIdxRange=[1]  outScalingMode=Treat bit field as an integer
  Real_Time_Command_Packet : etargetslib/Byte Unpack  dimensions={1, 1, 1, 1, 1, 1, 1, 1}  datatypes={'uint8', 'uint8', 'uint8', 'uint8', 'uint8', 'uint8', 'uint8', 'uint8'}  byteAlign=1
  Terminator{,1..7} (8 alike) : Terminator
  wires:
  Real_Time_Command_Packet/8 -> Terminator/1
  Real_Time_Command_Packet/7 -> Terminator1/1
  Real_Time_Command_Packet/6 -> Terminator2/1
  Real_Time_Command_Packet/5 -> Terminator3/1
  Real_Time_Command_Packet/4 -> Terminator4/1
  Real_Time_Command_Packet/3 -> Terminator5/1
  Real_Time_Command_Packet/2 -> Terminator6/1
  Length/1 -> Terminator7/1
  Data/1 -> Real_Time_Command_Packet/1
  Real_Time_Command_Packet/1 -> Extract Bits1/1, Extract Bits/1
  Extract Bits/1 -> Data Store Write1/1
  Extract Bits1/1 -> Data Store Write/1

== system CAN_TX_RX/Tx Event Based BMS Identification Packets (Send to VCU)   /BMS_FW_Version ==
  Byte1 : Inport
  FW_Version_Bytes : Inport  Port=2
  Byte Pack : etargetslib/Byte Pack  datatypes={'uint32'}  byteAlign=1
  Mux : Mux  Inputs=2
  BMS_SerialNo_FW_Version : Outport
  wires:
  Byte Pack/1 -> Mux/2  "Byte13_16"
  Byte1/1 -> Mux/1
  FW_Version_Bytes/1 -> Byte Pack/1
  Mux/1 -> BMS_SerialNo_FW_Version/1

== system CAN_TX_RX/Tx Event Based BMS Identification Packets (Send to VCU)   /BMS_SerialNo_Packet1 ==
  Byte1: 4 : Inport
  Byte5: 8 : Inport  Port=2
  Byte Pack : etargetslib/Byte Pack  datatypes={'uint32'}  byteAlign=1
  Byte Pack1 : etargetslib/Byte Pack  datatypes={'uint32'}  byteAlign=1
  Mux : Mux  Inputs=2
  BMS_SerialNo : Outport
  wires:
  Mux/1 -> BMS_SerialNo/1
  Byte Pack1/1 -> Mux/1  "Byte1_4"
  Byte Pack/1 -> Mux/2  "Byte5_8"
  Byte1: 4/1 -> Byte Pack1/1
  Byte5: 8/1 -> Byte Pack/1

== system CAN_TX_RX/Tx Event Based BMS Identification Packets (Send to VCU)   /BMS_SerialNo_Packet2 ==
  Byte1: 4 : Inport
  Byte5: 8 : Inport  Port=2
  Byte Pack : etargetslib/Byte Pack  datatypes={'uint32'}  byteAlign=1
  Byte Pack1 : etargetslib/Byte Pack  datatypes={'uint32'}  byteAlign=1
  Mux : Mux  Inputs=2
  BMS_SerialNo : Outport
  wires:
  Byte5: 8/1 -> Byte Pack/1
  Byte1: 4/1 -> Byte Pack1/1
  Byte Pack/1 -> Mux/2  "Byte13_16"
  Byte Pack1/1 -> Mux/1  "Byte9_12"
  Mux/1 -> BMS_SerialNo/1

== system CAN_TX_RX/Tx Event Based BMS Identification Packets (Send to VCU)   /Tx Successful ==
  Action Port : ActionPort  ActionPortLabel=if(u1 == 1 & u2 == 1 & u3 == 1)
  Cast To Boolean : DataTypeConversion  OutDataTypeStr=boolean
  Counter Limited : simulink/Sources/Counter Limited  uplimit=1  tsamp=-1
  Digital_Output : mbd_s32k1xx_ec_toolbox/GPIO Blocks/Digital_Output  gpio_pin=PTD0: [PTD0 | Port D I/O]  init_val=High  drive_strength=Low
  wires:
  Counter Limited/1 -> Cast To Boolean/1
  Cast To Boolean/1 -> Digital_Output/1

== system CAN_TX_RX/Tx Event Based Real Time Command Packet (Send to OBC)/Tx Successful ==
  Action Port : ActionPort  ActionPortLabel=if(u1 == 1)
  Blue_LED : mbd_s32k1xx_ec_toolbox/GPIO Blocks/Digital_Output  gpio_pin=PTD0: [PTD0 | Port D I/O]  init_val=High  drive_strength=Low
  Cast To Boolean : DataTypeConversion  OutDataTypeStr=boolean
  Counter Limited : simulink/Sources/Counter Limited  uplimit=1  tsamp=-1
  wires:
  Counter Limited/1 -> Cast To Boolean/1
  Cast To Boolean/1 -> Blue_LED/1

== system CAN_TX_RX/Tx Event Based Status Packets 5 ~ 14 (Send to VCU)/Status_Packet5 ==
  Data Store Memory : DataStoreMemory  DataStoreName=Byte1  ReadBeforeWriteMsg=warning  WriteAfterWriteMsg=warning  WriteAfterReadMsg=warning  ShowAdditionalParam=off  OutDataTypeStr=uint8
  Data Store Memory1 : DataStoreMemory  DataStoreName=Byte2  ReadBeforeWriteMsg=warning  WriteAfterWriteMsg=warning  WriteAfterReadMsg=warning  ShowAdditionalParam=off  OutDataTypeStr=uint8
  Grouping Data : Subsystem
  Packing Data : Subsystem
  Packet5 : Outport
  wires:
  Grouping Data/1(Packet5) -> Packet5/1

== system CAN_TX_RX/Tx Event Based Status Packets 5 ~ 14 (Send to VCU)/Status_Packet6 ==
  Data Store Memory : DataStoreMemory  DataStoreName=Byte1_2  ReadBeforeWriteMsg=warning  WriteAfterWriteMsg=warning  WriteAfterReadMsg=warning  ShowAdditionalParam=off  OutDataTypeStr=uint16
  Data Store Memory1 : DataStoreMemory  DataStoreName=Byte3_4  ReadBeforeWriteMsg=warning  WriteAfterWriteMsg=warning  WriteAfterReadMsg=warning  ShowAdditionalParam=off  OutDataTypeStr=uint16
  Data Store Memory2 : DataStoreMemory  DataStoreName=Byte5_6  ReadBeforeWriteMsg=warning  WriteAfterWriteMsg=warning  WriteAfterReadMsg=warning  ShowAdditionalParam=off  OutDataTypeStr=uint16
  Data Store Memory3 : DataStoreMemory  DataStoreName=Byte7_8  ReadBeforeWriteMsg=warning  WriteAfterWriteMsg=warning  WriteAfterReadMsg=warning  ShowAdditionalParam=off  OutDataTypeStr=uint16
  Grouping Data : Subsystem
  Packing Data : Subsystem
  Packet6 : Outport
  wires:
  Grouping Data/1(Packet6) -> Packet6/1

== system CAN_TX_RX/Tx Event Based Status Packets 5 ~ 14 (Send to VCU)/Tx Successful ==
  Action Port : ActionPort
  Cast To Boolean : DataTypeConversion  OutDataTypeStr=boolean
  Counter Limited : simulink/Sources/Counter Limited  uplimit=1  tsamp=-1
  Digital_Output : mbd_s32k1xx_ec_toolbox/GPIO Blocks/Digital_Output  gpio_pin=PTD0: [PTD0 | Port D I/O]  init_val=High  drive_strength=Low
  wires:
  Cast To Boolean/1 -> Digital_Output/1
  Counter Limited/1 -> Cast To Boolean/1

== system CAN_TX_RX/Tx every 100ms (Send to VCU)/Status_Packet4 ==
  Data Store Memory : DataStoreMemory  DataStoreName=Byte1  ReadBeforeWriteMsg=warning  WriteAfterWriteMsg=warning  WriteAfterReadMsg=warning  ShowAdditionalParam=off  OutDataTypeStr=uint8
  Data Store Memory1 : DataStoreMemory  DataStoreName=Byte2  ReadBeforeWriteMsg=warning  WriteAfterWriteMsg=warning  WriteAfterReadMsg=warning  ShowAdditionalParam=off  OutDataTypeStr=uint8
  Data Store Memory2 : DataStoreMemory  DataStoreName=Byte3  ReadBeforeWriteMsg=warning  WriteAfterWriteMsg=warning  WriteAfterReadMsg=warning  ShowAdditionalParam=off  OutDataTypeStr=uint8
  Data Store Memory3 : DataStoreMemory  DataStoreName=Byte4  ReadBeforeWriteMsg=warning  WriteAfterWriteMsg=warning  WriteAfterReadMsg=warning  ShowAdditionalParam=off  OutDataTypeStr=uint8
  Data Store Memory5 : DataStoreMemory  DataStoreName=Byte8  ReadBeforeWriteMsg=warning  WriteAfterWriteMsg=warning  WriteAfterReadMsg=warning  ShowAdditionalParam=off  OutDataTypeStr=uint8
  Data Store Memory6 : DataStoreMemory  DataStoreName=Byte5  ReadBeforeWriteMsg=warning  WriteAfterWriteMsg=warning  WriteAfterReadMsg=warning  ShowAdditionalParam=off  OutDataTypeStr=uint8
  Data Store Memory7 : DataStoreMemory  DataStoreName=Byte6  ReadBeforeWriteMsg=warning  WriteAfterWriteMsg=warning  WriteAfterReadMsg=warning  ShowAdditionalParam=off  OutDataTypeStr=uint8
  Data Store Memory8 : DataStoreMemory  DataStoreName=Byte7  ReadBeforeWriteMsg=warning  WriteAfterWriteMsg=warning  WriteAfterReadMsg=warning  ShowAdditionalParam=off  OutDataTypeStr=uint8
  Grouping Data : Subsystem
  Packing Data : Subsystem
  Packet4 : Outport
  wires:
  Grouping Data/1(Packet4) -> Packet4/1

== system CAN_TX_RX/Tx every 100ms (Send to VCU)/Tx Succesful ==
  Action Port : ActionPort  ActionPortLabel=if(u1 == 1)
  Cast To Boolean : DataTypeConversion  OutDataTypeStr=boolean
  Counter Limited : simulink/Sources/Counter Limited  uplimit=1  tsamp=-1
  Green_LED : mbd_s32k1xx_ec_toolbox/GPIO Blocks/Digital_Output  gpio_pin=PTD16: [PTD16 | Port D I/O]  init_val=High  drive_strength=Low
  wires:
  Cast To Boolean/1 -> Green_LED/1
  Counter Limited/1 -> Cast To Boolean/1

== system CAN_TX_RX/Tx every 200ms (Send to VCU)/Status_Packet2 ==
  Data Store Memory : DataStoreMemory  DataStoreName=Byte1_2  ReadBeforeWriteMsg=warning  WriteAfterWriteMsg=warning  WriteAfterReadMsg=warning  ShowAdditionalParam=off  OutDataTypeStr=uint16
  Data Store Memory2 : DataStoreMemory  DataStoreName=Byte3_4  ReadBeforeWriteMsg=warning  WriteAfterWriteMsg=warning  WriteAfterReadMsg=warning  ShowAdditionalParam=off  OutDataTypeStr=uint16
  Data Store Memory7 : DataStoreMemory  DataStoreName=Byte5_6  ReadBeforeWriteMsg=warning  WriteAfterWriteMsg=warning  WriteAfterReadMsg=warning  ShowAdditionalParam=off  OutDataTypeStr=uint16
  Data Store Memory9 : DataStoreMemory  DataStoreName=Byte7_8  ReadBeforeWriteMsg=warning  WriteAfterWriteMsg=warning  WriteAfterReadMsg=warning  ShowAdditionalParam=off  OutDataTypeStr=uint16
  Grouping Data : Subsystem
  Packing Data : Subsystem
  Packet2 : Outport
  wires:
  Grouping Data/1(Packet2) -> Packet2/1

== system CAN_TX_RX/Tx every 200ms (Send to VCU)/Status_Packet3 ==
  Data Store Memory : DataStoreMemory  DataStoreName=Byte1  ReadBeforeWriteMsg=warning  WriteAfterWriteMsg=warning  WriteAfterReadMsg=warning  ShowAdditionalParam=off  OutDataTypeStr=uint8
  Data Store Memory1 : DataStoreMemory  DataStoreName=Byte2  ReadBeforeWriteMsg=warning  WriteAfterWriteMsg=warning  WriteAfterReadMsg=warning  ShowAdditionalParam=off  OutDataTypeStr=uint8
  Data Store Memory2 : DataStoreMemory  DataStoreName=Byte3  ReadBeforeWriteMsg=warning  WriteAfterWriteMsg=warning  WriteAfterReadMsg=warning  ShowAdditionalParam=off  OutDataTypeStr=uint8
  Data Store Memory3 : DataStoreMemory  DataStoreName=Byte4  ReadBeforeWriteMsg=warning  WriteAfterWriteMsg=warning  WriteAfterReadMsg=warning  ShowAdditionalParam=off  OutDataTypeStr=uint8
  Data Store Memory4 : DataStoreMemory  DataStoreName=Byte7  ReadBeforeWriteMsg=warning  WriteAfterWriteMsg=warning  WriteAfterReadMsg=warning  ShowAdditionalParam=off  OutDataTypeStr=uint8
  Data Store Memory5 : DataStoreMemory  DataStoreName=Byte8  ReadBeforeWriteMsg=warning  WriteAfterWriteMsg=warning  WriteAfterReadMsg=warning  ShowAdditionalParam=off  OutDataTypeStr=uint8
  Data Store Memory9 : DataStoreMemory  DataStoreName=Byte5_6  ReadBeforeWriteMsg=warning  WriteAfterWriteMsg=warning  WriteAfterReadMsg=warning  ShowAdditionalParam=off  OutDataTypeStr=uint16
  Grouping Data : Subsystem
  Packing Data : Subsystem
  Packet3 : Outport
  wires:
  Grouping Data/1(Packet3) -> Packet3/1

== system CAN_TX_RX/Tx every 200ms (Send to VCU)/Tx Successful ==
  Action Port : ActionPort  ActionPortLabel=if(u1 == 1 & u2 == 1)
  Blue_LED : mbd_s32k1xx_ec_toolbox/GPIO Blocks/Digital_Output  gpio_pin=PTD0: [PTD0 | Port D I/O]  init_val=High  drive_strength=Low
  Cast To Boolean : DataTypeConversion  OutDataTypeStr=boolean
  Counter Limited : simulink/Sources/Counter Limited  uplimit=1  tsamp=-1
  wires:
  Counter Limited/1 -> Cast To Boolean/1
  Cast To Boolean/1 -> Blue_LED/1

== system CAN_TX_RX/Tx every 50ms (Send to VCU)/Status_Packet1 ==
  Data Store Memory : DataStoreMemory  DataStoreName=Byte1  ReadBeforeWriteMsg=warning  WriteAfterWriteMsg=warning  WriteAfterReadMsg=warning  ShowAdditionalParam=off  OutDataTypeStr=uint8
  Data Store Memory1 : DataStoreMemory  DataStoreName=Byte2  ReadBeforeWriteMsg=warning  WriteAfterWriteMsg=warning  WriteAfterReadMsg=warning  ShowAdditionalParam=off  OutDataTypeStr=uint8
  Data Store Memory2 : DataStoreMemory  DataStoreName=Byte3  ReadBeforeWriteMsg=warning  WriteAfterWriteMsg=warning  WriteAfterReadMsg=warning  ShowAdditionalParam=off  OutDataTypeStr=uint8
  Data Store Memory3 : DataStoreMemory  DataStoreName=Byte4_5  ReadBeforeWriteMsg=warning  WriteAfterWriteMsg=warning  WriteAfterReadMsg=warning  ShowAdditionalParam=off  OutDataTypeStr=uint16
  Data Store Memory4 : DataStoreMemory  DataStoreName=Byte6_7  ReadBeforeWriteMsg=warning  WriteAfterWriteMsg=warning  WriteAfterReadMsg=warning  ShowAdditionalParam=off  OutDataTypeStr=uint16
  Data Store Memory5 : DataStoreMemory  DataStoreName=Byte8  ReadBeforeWriteMsg=warning  WriteAfterWriteMsg=warning  WriteAfterReadMsg=warning  ShowAdditionalParam=off  OutDataTypeStr=uint8
  Grouping Data : Subsystem
  Packing Data : Subsystem
  Packet1 : Outport
  wires:
  Grouping Data/1(Packet1) -> Packet1/1

== system CAN_TX_RX/Tx every 50ms (Send to VCU)/Tx Succesful ==
  Action Port : ActionPort  ActionPortLabel=if(u1 == 1)
  Cast To Boolean : DataTypeConversion  OutDataTypeStr=boolean
  Counter Limited : simulink/Sources/Counter Limited  uplimit=1  tsamp=-1
  Red_LED : mbd_s32k1xx_ec_toolbox/GPIO Blocks/Digital_Output  gpio_pin=PTD15: [PTD15 | Port D I/O]  init_val=High  drive_strength=Low
  wires:
  Counter Limited/1 -> Cast To Boolean/1
  Cast To Boolean/1 -> Red_LED/1

== system CAN_TX_RX/Tx Event Based Status Packets 5 ~ 14 (Send to VCU)/Status_Packet5/Grouping Data ==
  Data Store Read6 : DataStoreRead  DataStoreName=Byte1
  Data Store Read7 : DataStoreRead  DataStoreName=Byte2
  Mux : Mux  Inputs=2
  Packet5 : Outport
  wires:
  Mux/1 -> Packet5/1
  Data Store Read6/1 -> Mux/1
  Data Store Read7/1 -> Mux/2

== system CAN_TX_RX/Tx Event Based Status Packets 5 ~ 14 (Send to VCU)/Status_Packet5/Packing Data ==
  Bit 1 : Constant  Value=5  OutDataTypeStr=uint8
  Bit 1:2 : Constant  Value=5  OutDataTypeStr=uint8
  Bit 2 : Constant  Value=5  OutDataTypeStr=uint8
  Bitwise OR : simulink/Logic and Bit Operations/Bitwise Operator  logicop=OR  UseBitMask=off  NumInputPorts=2  BitMask=bin2dec('11011001')  BitMaskRealWorld=Stored Integer
  DEVICE_INFO_SELECTION : DataStoreWrite  DataStoreName=Byte1
  DISABLE_CHARGING_DC_DC_ENABLED : DataStoreWrite  DataStoreName=Byte2
  Shift Arithmetic : ArithShift  BitShiftNumber=-6
  Shift Arithmetic1 : ArithShift  BitShiftNumber=-7
  Shift Arithmetic2 : ArithShift  BitShiftNumber=-6
  wires:
  Bit 1:2/1 -> Shift Arithmetic/1
  Shift Arithmetic/1 -> DEVICE_INFO_SELECTION/1
  Shift Arithmetic1/1 -> Bitwise OR/1
  Shift Arithmetic2/1 -> Bitwise OR/2
  Bitwise OR/1 -> DISABLE_CHARGING_DC_DC_ENABLED/1
  Bit 1/1 -> Shift Arithmetic1/1
  Bit 2/1 -> Shift Arithmetic2/1

== system CAN_TX_RX/Tx Event Based Status Packets 5 ~ 14 (Send to VCU)/Status_Packet6/Grouping Data ==
  Byte Pack1 : etargetslib/Byte Pack  datatypes={'uint16', 'uint16', 'uint16', 'uint16'}  byteAlign=1
  Data Store Read : DataStoreRead  DataStoreName=Byte1_2
  Data Store Read1 : DataStoreRead  DataStoreName=Byte3_4
  Data Store Read2 : DataStoreRead  DataStoreName=Byte5_6
  Data Store Read3 : DataStoreRead  DataStoreName=Byte7_8
  Packet6 : Outport
  wires:
  Data Store Read/1 -> Byte Pack1/1
  Data Store Read1/1 -> Byte Pack1/2
  Data Store Read2/1 -> Byte Pack1/3
  Data Store Read3/1 -> Byte Pack1/4
  Byte Pack1/1 -> Packet6/1

== system CAN_TX_RX/Tx Event Based Status Packets 5 ~ 14 (Send to VCU)/Status_Packet6/Packing Data ==
  Constant : Constant  Value=12000  OutDataTypeStr=uint16
  Constant1 : Constant  Value=1289  OutDataTypeStr=uint16
  Constant2 : Constant  Value=45633  OutDataTypeStr=uint16
  Constant3 : Constant  OutDataTypeStr=uint16
  OVERVOLTAGE_ERROR_THRESHOLD : DataStoreWrite  DataStoreName=Byte1_2
  OVERVOLTAGE_WARNING_THRESHOLD : DataStoreWrite  DataStoreName=Byte3_4
  UNDERVOLTAGE_ERROR_THRESHOLD : DataStoreWrite  DataStoreName=Byte5_6
  UNDERVOLTAGE_WARNING_THRESHOLD : DataStoreWrite  DataStoreName=Byte7_8
  wires:
  Constant3/1 -> UNDERVOLTAGE_WARNING_THRESHOLD/1
  Constant2/1 -> UNDERVOLTAGE_ERROR_THRESHOLD/1
  Constant1/1 -> OVERVOLTAGE_WARNING_THRESHOLD/1
  Constant/1 -> OVERVOLTAGE_ERROR_THRESHOLD/1

== system CAN_TX_RX/Tx every 100ms (Send to VCU)/Status_Packet4/Grouping Data ==
  Data Store Read : DataStoreRead  DataStoreName=Byte1
  Data Store Read1 : DataStoreRead  DataStoreName=Byte2
  Data Store Read2 : DataStoreRead  DataStoreName=Byte3
  Data Store Read3 : DataStoreRead  DataStoreName=Byte4
  Data Store Read4 : DataStoreRead  DataStoreName=Byte5
  Data Store Read5 : DataStoreRead  DataStoreName=Byte6
  Data Store Read6 : DataStoreRead  DataStoreName=Byte7
  Data Store Read7 : DataStoreRead  DataStoreName=Byte8
  Mux : Mux  Inputs=8
  Packet4 : Outport
  wires:
  Mux/1 -> Packet4/1
  Data Store Read/1 -> Mux/1
  Data Store Read1/1 -> Mux/2
  Data Store Read2/1 -> Mux/3
  Data Store Read3/1 -> Mux/4
  Data Store Read4/1 -> Mux/5
  Data Store Read5/1 -> Mux/6
  Data Store Read6/1 -> Mux/7
  Data Store Read7/1 -> Mux/8
